simulink model "parallel_prediction_and_cost_function_6phase"  (R2022a)
settings: Solver=FixedStepDiscrete  StartTime=0.0  StopTime=10.0  RelTol=1e-3
undefined symbols (not defined in the file or in its folder): f_c, L_d, L_q, L_x, L_y, p, psi_pm, R_ph
libraries: hdlsllib x5
(part 1 of 3)
settings Model: DataTypeOverride=Off  Creator=Andre Merx  LastModifiedBy=Andre Merx
settings SolverCC: AlgebraicLoopSolver=TrustRegion
settings DataIOCC: LimitDataPoints=on  SaveOutput=off  SaveTime=off
settings OptimizationCC: BlockReduction=off  ConditionallyExecuteInputs=off  DefaultParameterBehavior=Inlined  LifeSpan=inf
settings DebuggingCC: AlgebraicLoopMsg=error  SingleTaskRateTransMsg=error  UnconnectedInputMsg=warning  UnconnectedOutputMsg=warning  UnconnectedLineMsg=warning  AllowSymbolicDim=off  StrictBusMsg=ErrorOnBusTreatedAsVector  SFUnexpectedBacktrackingDiag=warning  SFNoUnconditionalDefaultTransitionDiag=warning  SFExecutionAtInitializationDiag=none  SFMachineParentedDataDiag=warning  ArithmeticOperatorsInVariantConditions=warning
settings HardwareCC: ProdBitPerPointer=32  ProdBitPerSizeT=32  ProdBitPerPtrDiffT=32  ProdLargestAtomicFloat=None  ProdIntDivRoundTo=Undefined  ProdEndianess=Unspecified  ProdWordSize=32  ProdHWDeviceType=ASIC/FPGA->ASIC/FPGA  ProdEqTarget=off
settings SFSimCC: SimUseLocalCustomCode=off  CustomCodeUndefinedFunction=UseInterfaceOnly
settings RTWCC: RTWUseLocalCustomCode=off
settings CodeAppCC: StateflowObjectComments=on
settings GRTTargetCC: TargetLangStandard=C89/C90 (ANSI)
settings ConfigComp: CovScope=ReferencedModels  CovMetricSettings=dw  CovSaveCumulativeToWorkspaceVar=on  CovSaveSingleToWorkspaceVar=on  CovExternalEMLEnable=off  CovSFcnEnable=off

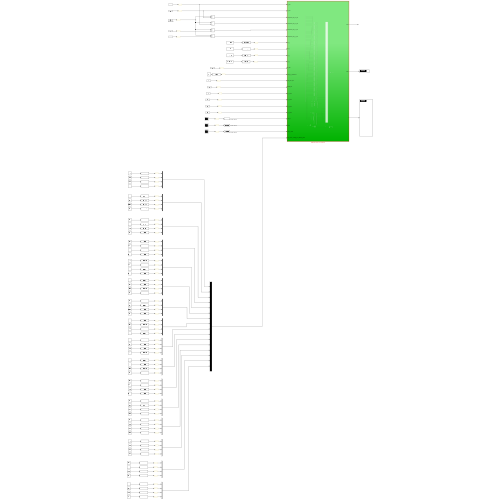
[thumbnail: Simulink's stored preview of the top-level diagram]
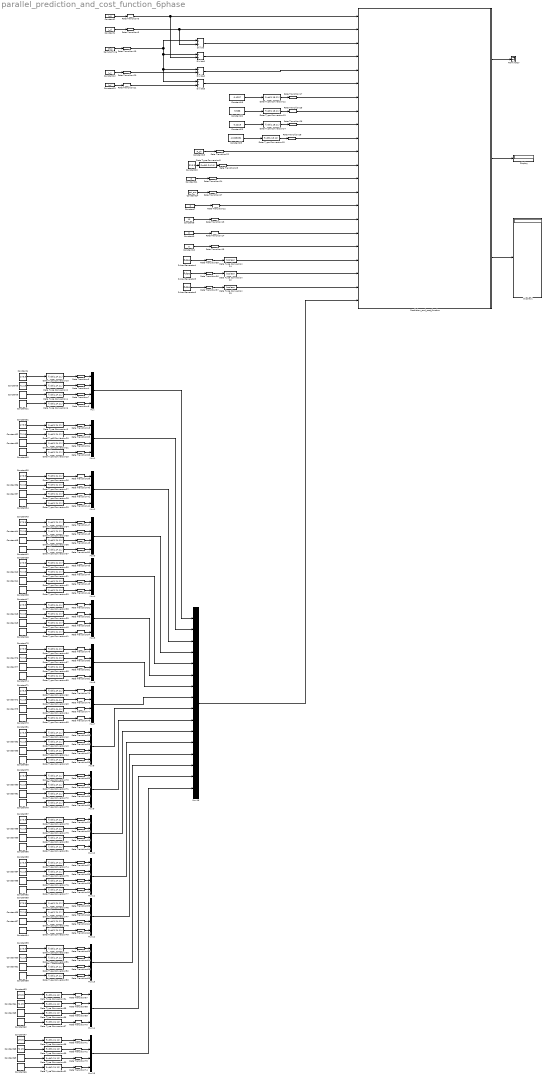
== system parallel_prediction_and_cost_function_6phase ==
  Constant1 : Constant  Value=L_d  OutDataTypeStr=single  SampleTime=-1
  Constant10 : Constant  Value=0  OutDataTypeStr=single  SampleTime=-1
  Constant{11,30,34,38,42,46,50,54,58,62,66,70,74,78,82,86} (16 alike) : Constant  Value=-163.1
  Constant12 : Constant  Value=L_x  OutDataTypeStr=single  SampleTime=-1
  Constant13 : Constant  Value=L_y  OutDataTypeStr=single  SampleTime=-1
  Constant18 : Constant  Value=0.4297
  Constant19 : Constant  Value=R_ph  OutDataTypeStr=single  SampleTime=-1
  Constant2 : Constant  Value=L_q  OutDataTypeStr=single  SampleTime=-1
  Constant20 : Constant  Value=313.3
  Constant21 : Constant  Value=p  OutDataTypeStr=single  SampleTime=-1
  Constant22 : Constant  Value=9.988
  Constant23 : Constant  Value=0.2219
  Constant24 : Constant  Value=psi_pm  OutDataTypeStr=single  SampleTime=-1
  Constant25 : Constant  Value=-0.003051
  Constant{4,31,35,39,43,47,51,55,59,63,67,71,75,79,83,87} (16 alike) : Constant  Value=173.9
  Constant{5,32,36,40,44,48,52,56,60,64,68,72,76,80,84,88} (16 alike) : Constant  Value=72.19
  Constant{6,33,37,41,45,49,53,57,61,65,69,73,77,81,85,89} (16 alike) : Constant  Value=-94.17
  Constant7 : Constant  Value=0  OutDataTypeStr=single  SampleTime=-1
  Constant8 : Constant  Value=10  OutDataTypeStr=single  SampleTime=-1
  Constant9 : Constant  Value=0  OutDataTypeStr=single  SampleTime=-1
  Data Type Conversion{2..6,10,20..21,25..81} (65 alike) : DataTypeConversion  OutDataTypeStr=fixdt(1,24,11)  SaturateOnIntegerOverflow=off  RndMeth=Floor
  Data Type Conversion{12..15} (4 alike) : DataTypeConversion  OutDataTypeStr=fixdt(1,18,11)  SaturateOnIntegerOverflow=off  RndMeth=Floor
  Data Type Conversion22 : DataTypeConversion  OutDataTypeStr=boolean  SaturateOnIntegerOverflow=off  RndMeth=Floor
  Data Type Conversion23 : DataTypeConversion  OutDataTypeStr=boolean  SaturateOnIntegerOverflow=off  RndMeth=Floor
  Data Type Conversion24 : DataTypeConversion  OutDataTypeStr=boolean  SaturateOnIntegerOverflow=off  RndMeth=Floor
  Display : Display
  Display1 : Display
  Divide{,1..3} (4 alike) : Product  Inputs=*/  RndMeth=Zero  SaturateOnIntegerOverflow=on
  Mux{,1..15} (16 alike) : Mux
  Mux16 : Mux  Inputs=16
  Prediction_and_cost_function : Subsystem  TreatAsAtomicUnit=on
  Pulse Generator4 : DiscretePulseGenerator  PulseType=Time based  Period=1/f_c
  Pulse Generator5 : DiscretePulseGenerator  PulseType=Time based  Period=1/f_c
  Pulse Generator6 : DiscretePulseGenerator  PulseType=Time based  Period=1/f_c
  Rate Transition{3..8,12..15,17..28,33..94} (84 alike) : RateTransition  OutPortSampleTime=Rt
  SampleTime : Constant  Value=1/f_c  OutDataTypeStr=single  SampleTime=-1
  Terminator : Terminator
  wires:
  Divide1/1 -> Prediction_and_cost_function/4(SampleTime_div_Lq_AXI)
  SampleTime/1 -> Rate Transition19/1
  Rate Transition20/1 -> Divide2/2
  Rate Transition19/1 -> Divide1/1, Divide3/1, Divide2/1, Divide/1
  Rate Transition21/1 -> Divide3/2
  Constant1/1 -> Rate Transition5/1
  Divide2/1 -> Prediction_and_cost_function/5(SampleTime_div_Lx_AXI)
  Data Type Conversion6/1 -> Rate Transition8/1
  Data Type Conversion10/1 -> Rate Transition3/1
  Divide/1 -> Prediction_and_cost_function/3(SampleTime_div_Ld_AXI)
  Constant9/1 -> Rate Transition14/1
  Constant13/1 -> Rate Transition21/1
  Data Type Conversion13/1 -> Rate Transition25/1
  Constant4/1 -> Data Type Conversion10/1
  Constant5/1 -> Data Type Conversion2/1
  Constant2/1 -> Rate Transition6/1
  Constant11/1 -> Data Type Conversion6/1
  Constant19/1 -> Rate Transition22/1
  Rate Transition25/1 -> Prediction_and_cost_function/8(iq_k_1)
  Constant23/1 -> Data Type Conversion14/1
  Constant21/1 -> Rate Transition24/1
  Constant12/1 -> Rate Transition20/1
  Data Type Conversion5/1 -> Rate Transition23/1
  Constant20/1 -> Data Type Conversion5/1
  Constant25/1 -> Data Type Conversion15/1
  Constant18/1 -> Data Type Conversion12/1
  Divide3/1 -> Prediction_and_cost_function/6(SampleTime_div_Ly_AXI)
  Constant7/1 -> Rate Transition12/1
  Data Type Conversion2/1 -> Rate Transition4/1
  Rate Transition5/1 -> Divide/2, Prediction_and_cost_function/2(Ld_AXI)
  Rate Transition26/1 -> Prediction_and_cost_function/9(ix_k_1)
  Data Type Conversion14/1 -> Rate Transition26/1
  Constant6/1 -> Data Type Conversion4/1
  Constant22/1 -> Data Type Conversion13/1
  Data Type Conversion4/1 -> Rate Transition7/1
  Constant8/1 -> Rate Transition13/1
  Constant10/1 -> Rate Transition15/1
  Rate Transition6/1 -> Divide1/2, Prediction_and_cost_function/1(Lq_AXI)
  Data Type Conversion15/1 -> Rate Transition28/1
  Constant24/1 -> Rate Transition27/1
  Data Type Conversion12/1 -> Rate Transition17/1
  Rate Transition17/1 -> Prediction_and_cost_function/7(id_k_1)
  Rate Transition28/1 -> Prediction_and_cost_function/10(iy_k_1)
  Rate Transition22/1 -> Prediction_and_cost_function/11(Rs_AXI)
  Rate Transition23/1 -> Prediction_and_cost_function/12(omega_m_measured)
  Rate Transition24/1 -> Prediction_and_cost_function/13(pole_pairs_AXI)
  Rate Transition27/1 -> Prediction_and_cost_function/14(psiPM_AXI)
  Rate Transition12/1 -> Prediction_and_cost_function/15(id_ref_AXI)
  Rate Transition13/1 -> Prediction_and_cost_function/16(iq_ref_AXI)
  Rate Transition14/1 -> Prediction_and_cost_function/17(ix_ref_AXI)
  Rate Transition15/1 -> Prediction_and_cost_function/18(iy_ref_AXI)
  Rate Transition37/1 -> Data Type Conversion23/1
  Pulse Generator6/1 -> Rate Transition37/1
  Data Type Conversion24/1 -> Prediction_and_cost_function/19(valid_in)  "curent_valid_in"
  Rate Transition36/1 -> Data Type Conversion22/1
  Data Type Conversion23/1 -> Prediction_and_cost_function/21(valid_in_ADC)  "curent_valid_in"
  Rate Transition35/1 -> Data Type Conversion24/1
  Pulse Generator5/1 -> Rate Transition36/1
  Data Type Conversion22/1 -> Prediction_and_cost_function/20(Reset)  "curent_valid_in"
  Pulse Generator4/1 -> Rate Transition35/1
  Data Type Conversion25/1 -> Rate Transition38/1
  Constant32/1 -> Data Type Conversion20/1
  Constant31/1 -> Data Type Conversion3/1
  Constant30/1 -> Data Type Conversion25/1
  Constant33/1 -> Data Type Conversion21/1
  Data Type Conversion21/1 -> Rate Transition34/1
  Data Type Conversion20/1 -> Rate Transition33/1
  Data Type Conversion3/1 -> Rate Transition18/1
  Data Type Conversion29/1 -> Rate Transition42/1
  Constant36/1 -> Data Type Conversion27/1
  Constant35/1 -> Data Type Conversion26/1
  Constant34/1 -> Data Type Conversion29/1
  Constant37/1 -> Data Type Conversion28/1
  Data Type Conversion28/1 -> Rate Transition41/1
  Data Type Conversion27/1 -> Rate Transition40/1
  Data Type Conversion26/1 -> Rate Transition39/1
  Data Type Conversion33/1 -> Rate Transition46/1
  Constant40/1 -> Data Type Conversion31/1
  Constant39/1 -> Data Type Conversion30/1
  Constant38/1 -> Data Type Conversion33/1
  Constant41/1 -> Data Type Conversion32/1
  Data Type Conversion32/1 -> Rate Transition45/1
  Data Type Conversion31/1 -> Rate Transition44/1
  Data Type Conversion30/1 -> Rate Transition43/1
  Data Type Conversion37/1 -> Rate Transition50/1
  Constant44/1 -> Data Type Conversion35/1
  Constant43/1 -> Data Type Conversion34/1
  Constant42/1 -> Data Type Conversion37/1
  Constant45/1 -> Data Type Conversion36/1
  Data Type Conversion36/1 -> Rate Transition49/1
  Data Type Conversion35/1 -> Rate Transition48/1
  Data Type Conversion34/1 -> Rate Transition47/1
  Data Type Conversion41/1 -> Rate Transition54/1
  Constant48/1 -> Data Type Conversion39/1
  Constant47/1 -> Data Type Conversion38/1
  Constant46/1 -> Data Type Conversion41/1
  Constant49/1 -> Data Type Conversion40/1
  Data Type Conversion40/1 -> Rate Transition53/1
  Data Type Conversion39/1 -> Rate Transition52/1
  Data Type Conversion38/1 -> Rate Transition51/1
  Data Type Conversion45/1 -> Rate Transition58/1
  Constant52/1 -> Data Type Conversion43/1
  Constant51/1 -> Data Type Conversion42/1
  Constant50/1 -> Data Type Conversion45/1
  Constant53/1 -> Data Type Conversion44/1
  Data Type Conversion44/1 -> Rate Transition57/1
  Data Type Conversion43/1 -> Rate Transition56/1
  Data Type Conversion42/1 -> Rate Transition55/1
  Data Type Conversion49/1 -> Rate Transition62/1
  Constant56/1 -> Data Type Conversion47/1
  Constant55/1 -> Data Type Conversion46/1
  Constant54/1 -> Data Type Conversion49/1
  Constant57/1 -> Data Type Conversion48/1
  Data Type Conversion48/1 -> Rate Transition61/1
  Data Type Conversion47/1 -> Rate Transition60/1
  Data Type Conversion46/1 -> Rate Transition59/1
  Data Type Conversion65/1 -> Rate Transition78/1
  Constant72/1 -> Data Type Conversion63/1
  Constant71/1 -> Data Type Conversion62/1
  Constant70/1 -> Data Type Conversion65/1
  Constant73/1 -> Data Type Conversion64/1
  Data Type Conversion64/1 -> Rate Transition77/1
  Data Type Conversion63/1 -> Rate Transition76/1
  Data Type Conversion62/1 -> Rate Transition75/1
  Data Type Conversion69/1 -> Rate Transition82/1
  Constant76/1 -> Data Type Conversion67/1
  Constant75/1 -> Data Type Conversion66/1
  Constant74/1 -> Data Type Conversion69/1
  Constant77/1 -> Data Type Conversion68/1
  Data Type Conversion68/1 -> Rate Transition81/1
  Data Type Conversion67/1 -> Rate Transition80/1
  Data Type Conversion66/1 -> Rate Transition79/1
  Data Type Conversion73/1 -> Rate Transition86/1
  Constant80/1 -> Data Type Conversion71/1
  Constant79/1 -> Data Type Conversion70/1
  Constant78/1 -> Data Type Conversion73/1
  Constant81/1 -> Data Type Conversion72/1
  Data Type Conversion72/1 -> Rate Transition85/1
  Data Type Conversion71/1 -> Rate Transition84/1
  Data Type Conversion70/1 -> Rate Transition83/1
  Data Type Conversion77/1 -> Rate Transition90/1
  Constant84/1 -> Data Type Conversion75/1
  Constant83/1 -> Data Type Conversion74/1
  Constant82/1 -> Data Type Conversion77/1
  Constant85/1 -> Data Type Conversion76/1
  Data Type Conversion76/1 -> Rate Transition89/1
  Data Type Conversion75/1 -> Rate Transition88/1
  Data Type Conversion74/1 -> Rate Transition87/1
  Data Type Conversion81/1 -> Rate Transition94/1
  Constant88/1 -> Data Type Conversion79/1
  Constant87/1 -> Data Type Conversion78/1
  Constant86/1 -> Data Type Conversion81/1
  Constant89/1 -> Data Type Conversion80/1
  Data Type Conversion80/1 -> Rate Transition93/1
  Data Type Conversion79/1 -> Rate Transition92/1
  Data Type Conversion78/1 -> Rate Transition91/1
  Data Type Conversion53/1 -> Rate Transition66/1
  Constant60/1 -> Data Type Conversion51/1
  Constant59/1 -> Data Type Conversion50/1
  Constant58/1 -> Data Type Conversion53/1
  Constant61/1 -> Data Type Conversion52/1
  Data Type Conversion52/1 -> Rate Transition65/1
  Data Type Conversion51/1 -> Rate Transition64/1
  Data Type Conversion50/1 -> Rate Transition63/1
  Data Type Conversion57/1 -> Rate Transition70/1
  Constant64/1 -> Data Type Conversion55/1
  Constant63/1 -> Data Type Conversion54/1
  Constant62/1 -> Data Type Conversion57/1
  Constant65/1 -> Data Type Conversion56/1
  Data Type Conversion56/1 -> Rate Transition69/1
  Data Type Conversion55/1 -> Rate Transition68/1
  Data Type Conversion54/1 -> Rate Transition67/1
  Data Type Conversion61/1 -> Rate Transition74/1
  Constant68/1 -> Data Type Conversion59/1
  Constant67/1 -> Data Type Conversion58/1
  Constant66/1 -> Data Type Conversion61/1
  Constant69/1 -> Data Type Conversion60/1
  Data Type Conversion60/1 -> Rate Transition73/1
  Data Type Conversion59/1 -> Rate Transition72/1
  Data Type Conversion58/1 -> Rate Transition71/1
  Rate Transition3/1 -> Mux/1
  Rate Transition4/1 -> Mux/2
  Rate Transition7/1 -> Mux/3
  Rate Transition8/1 -> Mux/4
  Rate Transition18/1 -> Mux1/1
  Rate Transition33/1 -> Mux1/2
  Rate Transition34/1 -> Mux1/3
  Rate Transition38/1 -> Mux1/4
  Rate Transition39/1 -> Mux2/1
  Rate Transition40/1 -> Mux2/2
  Rate Transition41/1 -> Mux2/3
  Rate Transition42/1 -> Mux2/4
  Rate Transition47/1 -> Mux3/1
  Rate Transition48/1 -> Mux3/2
  Rate Transition49/1 -> Mux3/3
  Rate Transition50/1 -> Mux3/4
  Rate Transition43/1 -> Mux4/1
  Rate Transition44/1 -> Mux4/2
  Rate Transition45/1 -> Mux4/3
  Rate Transition46/1 -> Mux4/4
  Rate Transition51/1 -> Mux5/1
  Rate Transition52/1 -> Mux5/2
  Rate Transition53/1 -> Mux5/3
  Rate Transition54/1 -> Mux5/4
  Rate Transition79/1 -> Mux6/1
  Rate Transition80/1 -> Mux6/2
  Rate Transition81/1 -> Mux6/3
  Rate Transition82/1 -> Mux6/4
  Rate Transition75/1 -> Mux7/1
  Rate Transition76/1 -> Mux7/2
  Rate Transition78/1 -> Mux7/4
  Rate Transition77/1 -> Mux7/3
  Rate Transition55/1 -> Mux8/1
  Rate Transition56/1 -> Mux8/2
  Rate Transition58/1 -> Mux8/4
  Rate Transition57/1 -> Mux8/3
  Rate Transition83/1 -> Mux9/1
  Rate Transition84/1 -> Mux9/2
  Rate Transition85/1 -> Mux9/3
  Rate Transition86/1 -> Mux9/4
  Rate Transition91/1 -> Mux10/1
  Rate Transition92/1 -> Mux10/2
  Rate Transition93/1 -> Mux10/3
  Rate Transition94/1 -> Mux10/4
  Rate Transition87/1 -> Mux11/1
  Rate Transition88/1 -> Mux11/2
  Rate Transition89/1 -> Mux11/3
  Rate Transition90/1 -> Mux11/4
  Rate Transition59/1 -> Mux12/1
  Rate Transition60/1 -> Mux12/2
  Rate Transition61/1 -> Mux12/3
  Rate Transition62/1 -> Mux12/4
  Rate Transition63/1 -> Mux13/1
  Rate Transition64/1 -> Mux13/2
  Rate Transition65/1 -> Mux13/3
  Rate Transition66/1 -> Mux13/4
  Rate Transition67/1 -> Mux14/1
  Rate Transition68/1 -> Mux14/2
  Rate Transition69/1 -> Mux14/3
  Rate Transition70/1 -> Mux14/4
  Rate Transition71/1 -> Mux15/1
  Rate Transition72/1 -> Mux15/2
  Rate Transition73/1 -> Mux15/3
  Rate Transition74/1 -> Mux15/4
  Mux/1 -> Mux16/1
  Mux1/1 -> Mux16/2
  Mux2/1 -> Mux16/3
  Mux3/1 -> Mux16/4
  Mux4/1 -> Mux16/5
  Mux5/1 -> Mux16/6
  Mux6/1 -> Mux16/7
  Mux7/1 -> Mux16/8
  Mux8/1 -> Mux16/9
  Mux9/1 -> Mux16/10
  Mux10/1 -> Mux16/11
  Mux11/1 -> Mux16/12
  Mux12/1 -> Mux16/13
  Mux13/1 -> Mux16/14
  Mux14/1 -> Mux16/15
  Mux15/1 -> Mux16/16
  Mux16/1 -> Prediction_and_cost_function/22(dqxy_phase_voltage_per_switching_state)
  Prediction_and_cost_function/2(Index) -> Display/1
  Prediction_and_cost_function/1(done) -> Terminator/1
  Prediction_and_cost_function/3(J) -> Display1/1

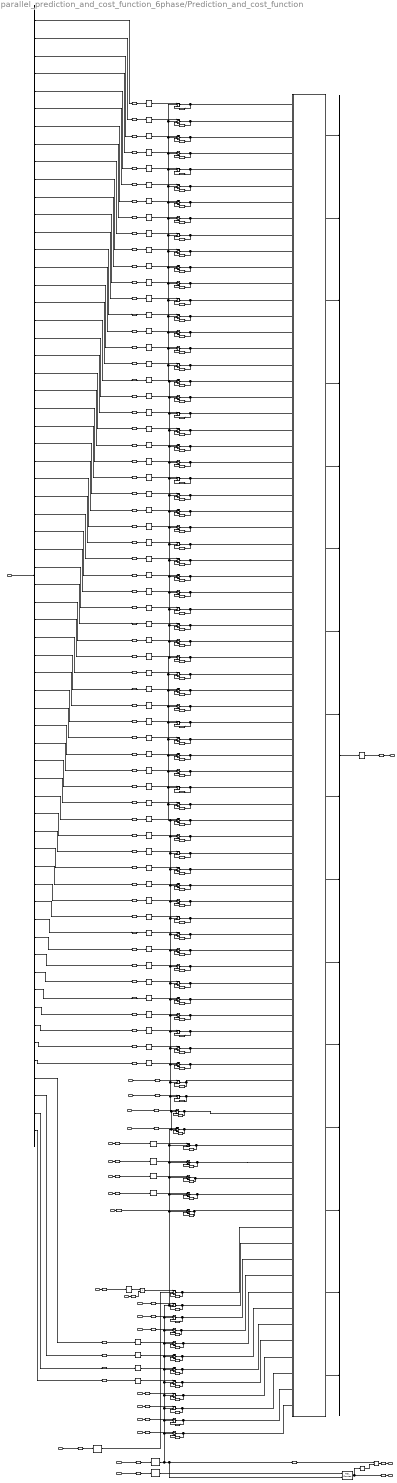
== system parallel_prediction_and_cost_function_6phase/Prediction_and_cost_function ==
  Lq_AXI : Inport
  Ld_AXI : Inport  Port=2
  SampleTime_div_Ld_AXI : Inport  Port=3
  SampleTime_div_Lq_AXI : Inport  Port=4
  SampleTime_div_Lx_AXI : Inport  Port=5
  SampleTime_div_Ly_AXI : Inport  Port=6
  id_k_1 : Inport  Port=7
  iq_k_1 : Inport  Port=8
  ix_k_1 : Inport  Port=9
  iy_k_1 : Inport  Port=10
  Rs_AXI : Inport  Port=11
  omega_m_measured : Inport  Port=12
  pole_pairs_AXI : Inport  Port=13
  psiPM_AXI : Inport  Port=14
  id_ref_AXI : Inport  Port=15
  iq_ref_AXI : Inport  Port=16
  ix_ref_AXI : Inport  Port=17
  iy_ref_AXI : Inport  Port=18
  valid_in : Inport  Port=19
  Reset : Inport  Port=20
  valid_in_ADC : Inport  Port=21
  dqxy_phase_voltage_per_switching_state : Inport  Port=22
  Compare To Constant : hdlsllib/Logic and Bit Operations/Compare To Constant  relop=<=  const=4  OutDataTypeStr=boolean
      settings: SourceProductBaseCode=SL
  Data Type Conversion{4,7..14,26..85} (69 alike) : DataTypeConversion  OutDataTypeStr=single  RndMeth=Nearest  SaturateOnIntegerOverflow=off
  Data Type Conversion18 : DataTypeConversion  OutDataTypeStr=fixdt(1,20,11)  RndMeth=Nearest  SaturateOnIntegerOverflow=off
  Delay{1..31,33..45,51,57,59..60,68,76..195} (169 alike) : Delay  DelayLength=1
  Delay58 : Delay  DelayLength=3
  Demux : Demux  Outputs=64
  Detect Rise Positive : hdlsllib/Logic and Bit Operations/Detect Rise Positive  vinit=0  OutDataTypeStr=boolean
      settings: SourceProductBaseCode=SL
  Detect Rise Positive1 : hdlsllib/Logic and Bit Operations/Detect Rise Positive  vinit=0  OutDataTypeStr=boolean
      settings: SourceProductBaseCode=SL
  Detect Rise Positive2 : hdlsllib/Logic and Bit Operations/Detect Rise Positive  vinit=0  OutDataTypeStr=boolean
      settings: SourceProductBaseCode=SL
  HDL Counter : hdlsllib/Sources/HDL Counter  CountType=Free running  CountInit=0  CountStep=1  CountMax=25  CountFromType=Initial value  CountFrom=0  CountResetPort=on  CountLoadPort=off  CountEnbPort=on  CountDirPort=off  CountHitOutputPort=off  CountDataType=Signed  CountWordLen=32  CountFracLen=0  CountSampTime=1
  Logical Operator : Logic  AllPortsSameDT=off  OutDataTypeStr=boolean
  Mux : Mux  Inputs=16
  Product : Product  Inputs=**
  Subsystem : Subsystem
  Switch_on{1..21,31..90} (81 alike) : Switch  Threshold=1  OutDataTypeStr=single  RndMeth=Simplest  SaturateOnIntegerOverflow=off  InputSameDT=off
  done : Outport
  Index : Outport  Port=2
  J : Outport  Port=3
  wires:
  Switch_on12/1 -> Subsystem/69(Rs15), Delay12/1
  Rs_AXI/1 -> Delay31/1
  Delay31/1 -> Switch_on12/1
  Delay23/1 -> Switch_on21/1
  Delay3/1 -> Switch_on3/3
  Delay10/1 -> Switch_on10/3
  Delay43/1 -> Switch_on2/1
  Switch_on5/1 -> Delay5/1, Subsystem/76(x_phase_voltage_per_switching_state15)
  Delay17/1 -> Switch_on18/3
  Switch_on10/1 -> Delay10/1, Subsystem/71(Lq15)
  Delay11/1 -> Switch_on11/3
  Switch_on6/1 -> Delay6/1, Subsystem/75(q_phase_voltage_per_switching_state15)
  Delay24/1 -> Switch_on20/1
  Delay36/1 -> Switch_on9/1
  Delay37/1 -> Switch_on8/1
  Delay1/1 -> Switch_on1/3
  Delay42/1 -> Switch_on3/1
  Product/1 -> Switch_on11/1  "omega_el"
  valid_in/1 -> Delay21/1
  Demux/64 -> Delay41/1
  Delay9/1 -> Switch_on9/3
  Data Type Conversion4/1 -> Product/1
  iy_k_1/1 -> Delay30/1
  Delay20/1 -> Switch_on21/3
  Delay35/1 -> Product/2
  pole_pairs_AXI/1 -> Delay35/1
  omega_m_measured/1 -> Delay51/1
  Switch_on18/1 -> Delay17/1, Subsystem/64(SampleTime_div_Ly15)
  Delay19/1 -> Switch_on20/3
  Delay13/1 -> Switch_on13/3
  Delay7/1 -> Switch_on7/3
  Delay4/1 -> Switch_on4/3
  Switch_on15/1 -> Delay14/1, Subsystem/67(ix_k_16)
  Delay18/1 -> Switch_on19/3
  Lq_AXI/1 -> Delay34/1
  Switch_on19/1 -> Delay18/1, Subsystem/63(SampleTime_div_Lx15)
  Switch_on20/1 -> Delay19/1, Subsystem/62(SampleTime_div_Lq15)
  Switch_on13/1 -> Delay13/1, Subsystem/68(iy_k_16)
  ix_k_1/1 -> Delay29/1
  Delay45/1 -> Switch_on14/1
  Delay2/1 -> Switch_on2/3
  Delay16/1 -> Switch_on17/3
  Switch_on17/1 -> Delay16/1, Subsystem/65(id_k_16)
  iq_k_1/1 -> Delay28/1
  Delay15/1 -> Switch_on16/3
  Switch_on16/1 -> Delay15/1, Subsystem/66(iq_k_16)
  Demux/61 -> Delay38/1
  iq_ref_AXI/1 -> Delay43/1
  Switch_on7/1 -> Delay7/1, Subsystem/74(d_phase_voltage_per_switching_state15)
  Switch_on11/1 -> Delay11/1, Subsystem/70(omega_el15)
  Delay33/1 -> Switch_on14/3
  Ld_AXI/1 -> Delay36/1
  Delay25/1 -> Switch_on19/1
  psiPM_AXI/1 -> Delay37/1
  Switch_on14/1 -> Delay33/1, Subsystem/81(iy_ref15)
  Delay12/1 -> Switch_on12/3
  Delay6/1 -> Switch_on6/3
  Delay21/1 -> Detect Rise Positive/1
  Switch_on3/1 -> Delay3/1, Subsystem/78(id_ref15)
  Switch_on21/1 -> Delay20/1, Subsystem/61(SampleTime_div_Ld15)
  Switch_on2/1 -> Delay2/1, Subsystem/79(iq_ref15)
  Delay34/1 -> Switch_on10/1
  Demux/62 -> Delay39/1
  iy_ref_AXI/1 -> Delay45/1
  Switch_on1/1 -> Delay1/1, Subsystem/80(ix_ref15)
  id_k_1/1 -> Delay27/1
  ix_ref_AXI/1 -> Delay44/1
  Switch_on9/1 -> Delay9/1, Subsystem/72(Ld15)
  Delay26/1 -> Switch_on18/1
  Demux/63 -> Delay40/1
  Delay14/1 -> Switch_on15/3
  Switch_on4/1 -> Delay4/1, Subsystem/77(y_phase_voltage_per_switching_state15)
  id_ref_AXI/1 -> Delay42/1
  Delay44/1 -> Switch_on1/1
  Switch_on8/1 -> Delay8/1, Subsystem/73(psiPM15)
  Delay5/1 -> Switch_on5/3
  Delay8/1 -> Switch_on8/3
  Delay27/1 -> Data Type Conversion7/1
  Delay28/1 -> Data Type Conversion8/1
  Delay29/1 -> Data Type Conversion9/1
  Delay30/1 -> Data Type Conversion10/1
  Delay51/1 -> Data Type Conversion4/1
  Delay38/1 -> Data Type Conversion11/1
  Delay39/1 -> Data Type Conversion12/1
  Delay40/1 -> Data Type Conversion13/1
  Delay41/1 -> Data Type Conversion14/1
  SampleTime_div_Ld_AXI/1 -> Delay23/1
  SampleTime_div_Lq_AXI/1 -> Delay24/1
  SampleTime_div_Lx_AXI/1 -> Delay25/1
  SampleTime_div_Ly_AXI/1 -> Delay26/1
  Data Type Conversion7/1 -> Switch_on17/1
  Data Type Conversion8/1 -> Switch_on16/1
  Data Type Conversion9/1 -> Switch_on15/1
  Data Type Conversion10/1 -> Switch_on13/1
  Data Type Conversion11/1 -> Switch_on7/1
  Data Type Conversion12/1 -> Switch_on6/1
  Data Type Conversion13/1 -> Switch_on5/1
  Data Type Conversion14/1 -> Switch_on4/1
  Reset/1 -> Delay57/1
  Delay57/1 -> Detect Rise Positive1/1
  Detect Rise Positive1/1 -> HDL Counter/1  "End_Cycle"
  HDL Counter/1 -> Compare To Constant/1, Delay59/1
  Logical Operator/1 -> Delay58/1
  Compare To Constant/1 -> Logical Operator/2
  Delay58/1 -> done/1
  Delay59/1 -> Index/1
  Delay22/1 -> Logical Operator/1
  valid_in_ADC/1 -> Delay60/1
  Detect Rise Positive2/1 -> Switch_on11/2  "End_Cycle"
  Delay60/1 -> Detect Rise Positive2/1
  Data Type Conversion18/1 -> Delay68/1
  Delay68/1 -> J/1
  Switch_on31/1 -> Subsystem/60(y_phase_voltage_per_switching_state14), Delay76/1
  Delay76/1 -> Switch_on31/3
  Switch_on32/1 -> Subsystem/59(x_phase_voltage_per_switching_state14), Delay77/1
  Delay77/1 -> Switch_on32/3
  Switch_on33/1 -> Subsystem/58(q_phase_voltage_per_switching_state14), Delay78/1
  Delay78/1 -> Switch_on33/3
  Switch_on34/1 -> Subsystem/57(d_phase_voltage_per_switching_state14), Delay79/1
  Delay79/1 -> Switch_on34/3
  Switch_on37/1 -> Subsystem/54(q_phase_voltage_per_switching_state13), Delay82/1
  Delay82/1 -> Switch_on37/3
  Delay83/1 -> Switch_on38/3
  Switch_on38/1 -> Subsystem/53(d_phase_voltage_per_switching_state13), Delay83/1
  Delay80/1 -> Switch_on35/3
  Switch_on35/1 -> Subsystem/56(y_phase_voltage_per_switching_state13), Delay80/1
  Delay81/1 -> Switch_on36/3
  Switch_on36/1 -> Subsystem/55(x_phase_voltage_per_switching_state13), Delay81/1
  Switch_on41/1 -> Subsystem/50(q_phase_voltage_per_switching_state12), Delay86/1
  Delay86/1 -> Switch_on41/3
  Delay87/1 -> Switch_on42/3
  Switch_on42/1 -> Subsystem/49(d_phase_voltage_per_switching_state12), Delay87/1
  Delay84/1 -> Switch_on39/3
  Switch_on39/1 -> Subsystem/52(y_phase_voltage_per_switching_state12), Delay84/1
  Delay85/1 -> Switch_on40/3
  Switch_on40/1 -> Subsystem/51(x_phase_voltage_per_switching_state12), Delay85/1
  Switch_on45/1 -> Subsystem/46(q_phase_voltage_per_switching_state11), Delay90/1
  Delay90/1 -> Switch_on45/3
  Delay91/1 -> Switch_on46/3
  Switch_on46/1 -> Subsystem/45(d_phase_voltage_per_switching_state11), Delay91/1
  Delay88/1 -> Switch_on43/3
  Switch_on43/1 -> Subsystem/48(y_phase_voltage_per_switching_state11), Delay88/1
  Delay89/1 -> Switch_on44/3
  Switch_on44/1 -> Subsystem/47(x_phase_voltage_per_switching_state11), Delay89/1
  Switch_on49/1 -> Subsystem/42(q_phase_voltage_per_switching_state10), Delay94/1
  Delay94/1 -> Switch_on49/3
  Delay95/1 -> Switch_on50/3
  Switch_on50/1 -> Subsystem/41(d_phase_voltage_per_switching_state10), Delay95/1
  Delay92/1 -> Switch_on47/3
  Switch_on47/1 -> Subsystem/44(y_phase_voltage_per_switching_state10), Delay92/1
  Delay93/1 -> Switch_on48/3
  Switch_on48/1 -> Subsystem/43(x_phase_voltage_per_switching_state10), Delay93/1
  Switch_on53/1 -> Subsystem/38(q_phase_voltage_per_switching_state9), Delay98/1
  Delay98/1 -> Switch_on53/3
  Delay99/1 -> Switch_on54/3
  Switch_on54/1 -> Subsystem/37(d_phase_voltage_per_switching_state9), Delay99/1
  Delay96/1 -> Switch_on51/3
  Switch_on51/1 -> Subsystem/40(y_phase_voltage_per_switching_state9), Delay96/1
  Delay97/1 -> Switch_on52/3
  Switch_on52/1 -> Subsystem/39(x_phase_voltage_per_switching_state9), Delay97/1
  Switch_on57/1 -> Subsystem/34(q_phase_voltage_per_switching_state8), Delay102/1
  Delay102/1 -> Switch_on57/3
  Delay103/1 -> Switch_on58/3
  Switch_on58/1 -> Subsystem/33(d_phase_voltage_per_switching_state8), Delay103/1
  Delay100/1 -> Switch_on55/3
  Switch_on55/1 -> Subsystem/36(y_phase_voltage_per_switching_state8), Delay100/1
  Delay101/1 -> Switch_on56/3
  Switch_on56/1 -> Subsystem/35(x_phase_voltage_per_switching_state8), Delay101/1
  Switch_on61/1 -> Subsystem/30(q_phase_voltage_per_switching_state7), Delay106/1
  Delay106/1 -> Switch_on61/3
  Delay107/1 -> Switch_on62/3
  Switch_on62/1 -> Subsystem/29(d_phase_voltage_per_switching_state7), Delay107/1
  Delay104/1 -> Switch_on59/3
  Switch_on59/1 -> Subsystem/32(y_phase_voltage_per_switching_state7), Delay104/1
  Delay105/1 -> Switch_on60/3
  Switch_on60/1 -> Subsystem/31(x_phase_voltage_per_switching_state7), Delay105/1
  Switch_on65/1 -> Subsystem/26(q_phase_voltage_per_switching_state6), Delay110/1
  Delay110/1 -> Switch_on65/3
  Delay111/1 -> Switch_on66/3
  Switch_on66/1 -> Subsystem/25(d_phase_voltage_per_switching_state6), Delay111/1
  Delay108/1 -> Switch_on63/3
  Switch_on63/1 -> Subsystem/28(y_phase_voltage_per_switching_state6), Delay108/1
  Delay109/1 -> Switch_on64/3
  Switch_on64/1 -> Subsystem/27(x_phase_voltage_per_switching_state6), Delay109/1
  Switch_on69/1 -> Subsystem/22(q_phase_voltage_per_switching_state5), Delay114/1
  Delay114/1 -> Switch_on69/3
  Delay115/1 -> Switch_on70/3
  Switch_on70/1 -> Subsystem/21(d_phase_voltage_per_switching_state5), Delay115/1
  Delay112/1 -> Switch_on67/3
  Switch_on67/1 -> Subsystem/24(y_phase_voltage_per_switching_state5), Delay112/1
  Delay113/1 -> Switch_on68/3
  Switch_on68/1 -> Subsystem/23(x_phase_voltage_per_switching_state5), Delay113/1
  Switch_on73/1 -> Subsystem/18(q_phase_voltage_per_switching_state4), Delay118/1
  Delay118/1 -> Switch_on73/3
  Delay119/1 -> Switch_on74/3
  Switch_on74/1 -> Subsystem/17(d_phase_voltage_per_switching_state4), Delay119/1
  Delay116/1 -> Switch_on71/3
  Switch_on71/1 -> Subsystem/20(y_phase_voltage_per_switching_state4), Delay116/1
  Delay117/1 -> Switch_on72/3
  Switch_on72/1 -> Subsystem/19(x_phase_voltage_per_switching_state4), Delay117/1
  Switch_on77/1 -> Subsystem/14(q_phase_voltage_per_switching_state3), Delay122/1
  Delay122/1 -> Switch_on77/3
  Delay123/1 -> Switch_on78/3
  Switch_on78/1 -> Subsystem/13(d_phase_voltage_per_switching_state3), Delay123/1
  Delay120/1 -> Switch_on75/3
  Switch_on75/1 -> Subsystem/16(y_phase_voltage_per_switching_state3), Delay120/1
  Delay121/1 -> Switch_on76/3
  Switch_on76/1 -> Subsystem/15(x_phase_voltage_per_switching_state3), Delay121/1
  Switch_on81/1 -> Subsystem/10(q_phase_voltage_per_switching_state2), Delay126/1
  Delay126/1 -> Switch_on81/3
  Delay127/1 -> Switch_on82/3
  Switch_on82/1 -> Subsystem/9(d_phase_voltage_per_switching_state2), Delay127/1
  Delay124/1 -> Switch_on79/3
  Switch_on79/1 -> Subsystem/12(y_phase_voltage_per_switching_state2), Delay124/1
  Delay125/1 -> Switch_on80/3
  Switch_on80/1 -> Subsystem/11(x_phase_voltage_per_switching_state2), Delay125/1
  Switch_on85/1 -> Subsystem/6(q_phase_voltage_per_switching_state1), Delay130/1
  Delay130/1 -> Switch_on85/3
  Delay131/1 -> Switch_on86/3
  Switch_on86/1 -> Subsystem/5(d_phase_voltage_per_switching_state1), Delay131/1
  Delay128/1 -> Switch_on83/3
  Switch_on83/1 -> Subsystem/8(y_phase_voltage_per_switching_state1), Delay128/1
  Delay129/1 -> Switch_on84/3
  Switch_on84/1 -> Subsystem/7(x_phase_voltage_per_switching_state1), Delay129/1
  Delay137/1 -> Data Type Conversion84/1
  Switch_on89/1 -> Subsystem/2(q_phase_voltage_per_switching_state), Delay134/1
  Delay134/1 -> Switch_on89/3
  Delay135/1 -> Switch_on90/3
  Switch_on90/1 -> Subsystem/1(d_phase_voltage_per_switching_state), Delay135/1
  Delay136/1 -> Data Type Conversion85/1
  Delay132/1 -> Switch_on87/3
  Switch_on87/1 -> Subsystem/4(y_phase_voltage_per_switching_state), Delay132/1
  Delay133/1 -> Switch_on88/3
  Switch_on88/1 -> Subsystem/3(x_phase_voltage_per_switching_state), Delay133/1
  Detect Rise Positive/1 -> Delay22/1, HDL Counter/2, Switch_on14/2, Switch_on1/2, Switch_on5/2, Switch_on8/2, Switch_on9/2, Switch_on12/2, Switch_on20/2, Switch_on90/2, Switch_on89/2, Switch_on88/2, Switch_on87/2, Switch_on86/2, Switch_on85/2, Switch_on84/2, Switch_on83/2, Switch_on82/2, Switch_on81/2, Switch_on80/2, Switch_on79/2, Switch_on78/2, Switch_on77/2, Switch_on76/2, Switch_on75/2, Switch_on74/2, Switch_on73/2, Switch_on72/2, Switch_on71/2, Switch_on70/2, Switch_on69/2, Switch_on68/2, Switch_on67/2, Switch_on66/2, Switch_on65/2, Switch_on64/2, Switch_on63/2, Switch_on62/2, Switch_on61/2, Switch_on60/2, Switch_on59/2, Switch_on58/2, Switch_on57/2, Switch_on56/2, Switch_on55/2, Switch_on54/2, Switch_on53/2, Switch_on52/2, Switch_on51/2, Switch_on50/2, Switch_on49/2, Switch_on48/2, Switch_on47/2, Switch_on46/2, Switch_on45/2, Switch_on44/2, Switch_on43/2, Switch_on42/2, Switch_on41/2, Switch_on40/2, Switch_on39/2, Switch_on38/2, Switch_on37/2, Switch_on36/2, Switch_on35/2, Switch_on34/2, Switch_on33/2, Switch_on32/2, Switch_on31/2, Switch_on21/2, Switch_on19/2, Switch_on18/2, Switch_on17/2, Switch_on16/2, Switch_on15/2, Switch_on13/2, Switch_on10/2, Switch_on7/2, Switch_on6/2, Switch_on4/2, Switch_on3/2, Switch_on2/2  "End_Cycle"
  Delay138/1 -> Data Type Conversion83/1
  Delay139/1 -> Data Type Conversion82/1
  Delay140/1 -> Data Type Conversion81/1
  Delay141/1 -> Data Type Conversion80/1
  Delay143/1 -> Data Type Conversion78/1
  Delay142/1 -> Data Type Conversion79/1
  Delay144/1 -> Data Type Conversion77/1
  Delay145/1 -> Data Type Conversion76/1
  Delay147/1 -> Data Type Conversion74/1
  Delay146/1 -> Data Type Conversion75/1
  Delay148/1 -> Data Type Conversion73/1
  Delay149/1 -> Data Type Conversion72/1
  Delay151/1 -> Data Type Conversion70/1
  Delay150/1 -> Data Type Conversion71/1
  Delay152/1 -> Data Type Conversion69/1
  Delay153/1 -> Data Type Conversion68/1
  Delay155/1 -> Data Type Conversion66/1
  Delay154/1 -> Data Type Conversion67/1
  Delay156/1 -> Data Type Conversion65/1
  Delay157/1 -> Data Type Conversion64/1
  Delay159/1 -> Data Type Conversion62/1
  Delay158/1 -> Data Type Conversion63/1
  Delay160/1 -> Data Type Conversion61/1
  Delay161/1 -> Data Type Conversion60/1
  Delay163/1 -> Data Type Conversion58/1
  Delay162/1 -> Data Type Conversion59/1
  Delay164/1 -> Data Type Conversion57/1
  Delay165/1 -> Data Type Conversion56/1
  Delay167/1 -> Data Type Conversion54/1
  Delay166/1 -> Data Type Conversion55/1
  Delay168/1 -> Data Type Conversion53/1
  Delay169/1 -> Data Type Conversion52/1
  Delay171/1 -> Data Type Conversion50/1
  Delay170/1 -> Data Type Conversion51/1
  Delay172/1 -> Data Type Conversion49/1
  Delay173/1 -> Data Type Conversion48/1
  Delay175/1 -> Data Type Conversion46/1
  Delay174/1 -> Data Type Conversion47/1
  Delay176/1 -> Data Type Conversion45/1
  Delay177/1 -> Data Type Conversion44/1
  Delay179/1 -> Data Type Conversion42/1
  Delay178/1 -> Data Type Conversion43/1
  Delay180/1 -> Data Type Conversion41/1
  Delay181/1 -> Data Type Conversion40/1
  Delay183/1 -> Data Type Conversion38/1
  Delay182/1 -> Data Type Conversion39/1
  Delay184/1 -> Data Type Conversion37/1
  Delay185/1 -> Data Type Conversion36/1
  Delay187/1 -> Data Type Conversion34/1
  Delay186/1 -> Data Type Conversion35/1
  Delay188/1 -> Data Type Conversion33/1
  Delay189/1 -> Data Type Conversion32/1
  Delay191/1 -> Data Type Conversion30/1
  Delay190/1 -> Data Type Conversion31/1
  Delay192/1 -> Data Type Conversion29/1
  Delay193/1 -> Data Type Conversion28/1
  Delay195/1 -> Data Type Conversion26/1
  Delay194/1 -> Data Type Conversion27/1
  Data Type Conversion26/1 -> Switch_on31/1
  Data Type Conversion27/1 -> Switch_on32/1
  Data Type Conversion28/1 -> Switch_on33/1
  Data Type Conversion29/1 -> Switch_on34/1
  Data Type Conversion30/1 -> Switch_on35/1
  Data Type Conversion31/1 -> Switch_on36/1
  Data Type Conversion32/1 -> Switch_on37/1
  Data Type Conversion33/1 -> Switch_on38/1
  Data Type Conversion34/1 -> Switch_on39/1
  Data Type Conversion35/1 -> Switch_on40/1
  Data Type Conversion36/1 -> Switch_on41/1
  Data Type Conversion37/1 -> Switch_on42/1
  Data Type Conversion38/1 -> Switch_on43/1
  Data Type Conversion39/1 -> Switch_on44/1
  Data Type Conversion40/1 -> Switch_on45/1
  Data Type Conversion41/1 -> Switch_on46/1
  Data Type Conversion42/1 -> Switch_on47/1
  Data Type Conversion43/1 -> Switch_on48/1
  Data Type Conversion44/1 -> Switch_on49/1
  Data Type Conversion45/1 -> Switch_on50/1
  Data Type Conversion46/1 -> Switch_on51/1
  Data Type Conversion47/1 -> Switch_on52/1
  Data Type Conversion48/1 -> Switch_on53/1
  Data Type Conversion49/1 -> Switch_on54/1
  Data Type Conversion50/1 -> Switch_on55/1
  Data Type Conversion51/1 -> Switch_on56/1
  Data Type Conversion52/1 -> Switch_on57/1
  Data Type Conversion53/1 -> Switch_on58/1
  Data Type Conversion54/1 -> Switch_on59/1
  Data Type Conversion55/1 -> Switch_on60/1
  Data Type Conversion56/1 -> Switch_on61/1
  Data Type Conversion57/1 -> Switch_on62/1
  Data Type Conversion58/1 -> Switch_on63/1
  Data Type Conversion59/1 -> Switch_on64/1
  Data Type Conversion60/1 -> Switch_on65/1
  Data Type Conversion61/1 -> Switch_on66/1
  Data Type Conversion62/1 -> Switch_on67/1
  Data Type Conversion63/1 -> Switch_on68/1
  Data Type Conversion64/1 -> Switch_on69/1
  Data Type Conversion65/1 -> Switch_on70/1
  Data Type Conversion66/1 -> Switch_on71/1
  Data Type Conversion67/1 -> Switch_on72/1
  Data Type Conversion68/1 -> Switch_on73/1
  Data Type Conversion69/1 -> Switch_on74/1
  Data Type Conversion70/1 -> Switch_on75/1
  Data Type Conversion71/1 -> Switch_on76/1
  Data Type Conversion72/1 -> Switch_on77/1
  Data Type Conversion73/1 -> Switch_on78/1
  Data Type Conversion74/1 -> Switch_on79/1
  Data Type Conversion75/1 -> Switch_on80/1
  Data Type Conversion76/1 -> Switch_on81/1
  Data Type Conversion77/1 -> Switch_on82/1
  Data Type Conversion78/1 -> Switch_on83/1
  Data Type Conversion79/1 -> Switch_on84/1
  Data Type Conversion80/1 -> Switch_on85/1
  Data Type Conversion81/1 -> Switch_on86/1
  Data Type Conversion82/1 -> Switch_on87/1
  Data Type Conversion83/1 -> Switch_on88/1
  Data Type Conversion84/1 -> Switch_on89/1
  Data Type Conversion85/1 -> Switch_on90/1
  dqxy_phase_voltage_per_switching_state/1 -> Demux/1
  Demux/1 -> Delay136/1
  Demux/2 -> Delay137/1
  Demux/3 -> Delay138/1
  Demux/4 -> Delay139/1
  Demux/5 -> Delay140/1
  Demux/6 -> Delay141/1
  Demux/7 -> Delay142/1
  Demux/8 -> Delay143/1
  Demux/9 -> Delay144/1
  Demux/10 -> Delay145/1
  Demux/11 -> Delay146/1
  Demux/12 -> Delay147/1
  Demux/13 -> Delay148/1
  Demux/14 -> Delay149/1
  Demux/15 -> Delay150/1
  Demux/16 -> Delay151/1
  Demux/17 -> Delay152/1
  Demux/18 -> Delay153/1
  Demux/19 -> Delay154/1
  Demux/20 -> Delay155/1
  Demux/21 -> Delay156/1
  Demux/22 -> Delay157/1
  Demux/23 -> Delay158/1
  Demux/24 -> Delay159/1
  Demux/25 -> Delay160/1
  Demux/26 -> Delay161/1
  Demux/27 -> Delay162/1
  Demux/28 -> Delay163/1
  Demux/29 -> Delay164/1
  Demux/30 -> Delay165/1
  Demux/31 -> Delay166/1
  Demux/32 -> Delay167/1
  Demux/33 -> Delay168/1
  Demux/34 -> Delay169/1
  Demux/35 -> Delay170/1
  Demux/36 -> Delay171/1
  Demux/37 -> Delay172/1
  Demux/38 -> Delay173/1
  Demux/39 -> Delay174/1
  Demux/40 -> Delay175/1
  Demux/41 -> Delay176/1
  Demux/42 -> Delay177/1
  Demux/43 -> Delay178/1
  Demux/44 -> Delay179/1
  Demux/45 -> Delay180/1
  Demux/46 -> Delay181/1
  Demux/47 -> Delay182/1
  Demux/48 -> Delay183/1
  Demux/49 -> Delay184/1
  Demux/50 -> Delay185/1
  Demux/51 -> Delay186/1
  Demux/52 -> Delay187/1
  Demux/53 -> Delay188/1
  Demux/54 -> Delay189/1
  Demux/55 -> Delay190/1
  Demux/56 -> Delay191/1
  Demux/57 -> Delay192/1
  Demux/58 -> Delay193/1
  Demux/59 -> Delay194/1
  Demux/60 -> Delay195/1
  Subsystem/16(J15) -> Mux/16
  Subsystem/15(J14) -> Mux/15
  Subsystem/14(J13) -> Mux/14
  Subsystem/13(J12) -> Mux/13
  Subsystem/12(J11) -> Mux/12
  Subsystem/11(J10) -> Mux/11
  Subsystem/10(J9) -> Mux/10
  Subsystem/9(J8) -> Mux/9
  Subsystem/8(J7) -> Mux/8
  Subsystem/7(J6) -> Mux/7
  Subsystem/6(J5) -> Mux/6
  Subsystem/5(J4) -> Mux/5
  Subsystem/4(J3) -> Mux/4
  Subsystem/3(J2) -> Mux/3
  Subsystem/2(J1) -> Mux/2
  Subsystem/1(J) -> Mux/1
  Mux/1 -> Data Type Conversion18/1
